simulink model "Classical_method"  (R2021a)
settings: Solver=VariableStepAuto  StartTime=0.0  StopTime=1400  RelTol=1e-3
values from neighbouring files (symbols this model uses):
  B = 0.029    [project.m]
  J = 0.1    [project.m]
  ke = 0.6    [project.m]
  kt = 0.6    [project.m]
  La = 1e-3    (= 0.001)    [project.m]
  Ra = 1    [project.m]
settings Model: SimulationMode=rapid-accelerator  Creator=User  LastModifiedBy=User
settings DataIOCC: ReturnWorkspaceOutputs=off

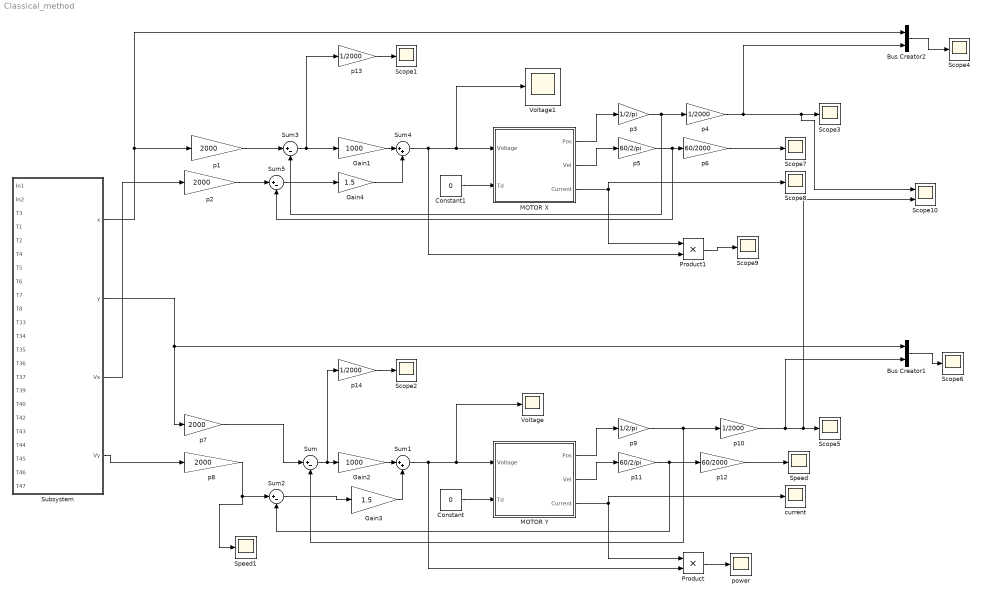
== system Classical_method ==
  Bus Creator1 : BusCreator  Inputs=2
  Bus Creator2 : BusCreator  Inputs=2
  Constant : Constant  Value=0
  Constant1 : Constant  Value=0
  Gain1 : Gain  Gain=1000
  Gain2 : Gain  Gain=1000
  Gain3 : Gain  Gain=1.5
  Gain4 : Gain  Gain=1.5
  MOTOR X : Subsystem
  MOTOR Y : Subsystem
  Product : Product
  Product1 : Product
  Scope{1..9} (9 alike) : Scope
  Scope10 : Scope  NumInputPorts=2
  Speed : Scope
  Speed1 : Scope
  Subsystem : Subsystem
  Sum{,2..3,5} (4 alike) : Sum  Inputs=|+-
  Sum1 : Sum  Inputs=|++
  Sum4 : Sum  Inputs=|++
  Voltage : Scope
  Voltage1 : Scope
  current : Scope
  p{1..2,7..8} (4 alike) : Gain  Gain=2000
  p{4,10,13..14} (4 alike) : Gain  Gain=1/2000
  p11 : Gain  Gain=60/2/pi
  p12 : Gain  Gain=60/2000
  p3 : Gain  Gain=1/2/pi
  p5 : Gain  Gain=60/2/pi
  p6 : Gain  Gain=60/2000
  p9 : Gain  Gain=1/2/pi
  power : Scope
  wires:
  MOTOR Y/1(Pos) -> p9/1
  p10/1 -> Bus Creator1/2, Scope10/2, Scope5/1
  Gain3/1 -> Sum1/2
  p5/1 -> Sum5/2, p6/1
  p7/1 -> Sum/1
  p3/1 -> Sum3/2, p4/1
  Constant1/1 -> MOTOR X/2(Td)
  MOTOR Y/3(Current) -> current/1, Product/1
  Sum5/1 -> Gain4/1
  Product1/1 -> Scope9/1
  Sum1/1 -> Product/2, Voltage/1, MOTOR Y/1(Voltage)
  p4/1 -> Bus Creator2/2, Scope10/1, Scope3/1
  Gain4/1 -> Sum4/2
  p12/1 -> Speed/1
  MOTOR X/3(Current) -> Scope8/1, Product1/1
  p8/1 -> Speed1/1, Sum2/1
  Bus Creator1/1 -> Scope6/1
  MOTOR X/2(Vel) -> p5/1
  Gain2/1 -> Sum1/1
  Gain1/1 -> Sum4/1
  Constant/1 -> MOTOR Y/2(Td)
  Product/1 -> power/1
  p6/1 -> Scope7/1
  Sum2/1 -> Gain3/1
  MOTOR Y/2(Vel) -> p11/1
  p2/1 -> Sum5/1
  Sum3/1 -> p13/1, Gain1/1
  p11/1 -> Sum2/2, p12/1
  Sum4/1 -> Product1/2, Voltage1/1, MOTOR X/1(Voltage)
  Sum/1 -> p14/1, Gain2/1
  Subsystem/2(y) -> Bus Creator1/1, p7/1
  Subsystem/3(Vx) -> p2/1
  p9/1 -> Sum/2, p10/1
  Subsystem/4(Vy) -> p8/1
  MOTOR X/1(Pos) -> p3/1
  Subsystem/1(x) -> p1/1, Bus Creator2/1
  Bus Creator2/1 -> Scope4/1
  p13/1 -> Scope1/1
  p14/1 -> Scope2/1
  p1/1 -> Sum3/1

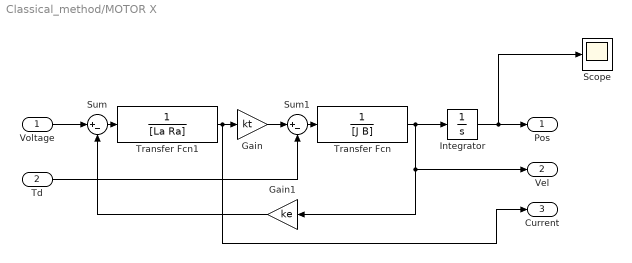
== system Classical_method/MOTOR X ==
  Voltage : Inport
  Td : Inport  Port=2
  Gain : Gain  Gain=kt
  Gain1 : Gain  Gain=ke
  Integrator : Integrator  InitialCondition=12000*pi
  Scope : Scope
  Sum : Sum  Inputs=|+-
  Sum1 : Sum  Inputs=|+-
  Transfer Fcn : TransferFcn  Denominator=[J B]
  Transfer Fcn1 : TransferFcn  Denominator=[La Ra]
  Pos : Outport  VectorParamsAs1DForOutWhenUnconnected=off
  Vel : Outport  Port=2  VectorParamsAs1DForOutWhenUnconnected=off
  Current : Outport  Port=3  VectorParamsAs1DForOutWhenUnconnected=off
  wires:
  Integrator/1 -> Scope/1, Pos/1
  Voltage/1 -> Sum/1
  Transfer Fcn/1 -> Integrator/1, Vel/1, Gain1/1
  Sum1/1 -> Transfer Fcn/1
  Td/1 -> Sum1/2
  Gain1/1 -> Sum/2
  Sum/1 -> Transfer Fcn1/1
  Transfer Fcn1/1 -> Current/1, Gain/1
  Gain/1 -> Sum1/1

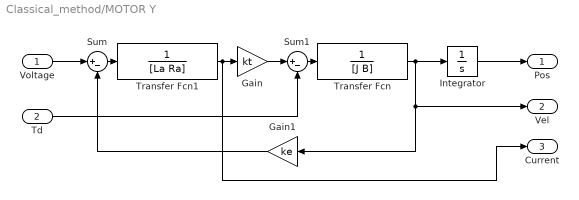
== system Classical_method/MOTOR Y ==
  Voltage : Inport
  Td : Inport  Port=2
  Gain : Gain  Gain=kt
  Gain1 : Gain  Gain=ke
  Integrator : Integrator  InitialCondition=8000*pi
  Sum : Sum  Inputs=|+-
  Sum1 : Sum  Inputs=|+-
  Transfer Fcn : TransferFcn  Denominator=[J B]
  Transfer Fcn1 : TransferFcn  Denominator=[La Ra]
  Pos : Outport  VectorParamsAs1DForOutWhenUnconnected=off
  Vel : Outport  Port=2  VectorParamsAs1DForOutWhenUnconnected=off
  Current : Outport  Port=3  VectorParamsAs1DForOutWhenUnconnected=off
  wires:
  Integrator/1 -> Pos/1
  Voltage/1 -> Sum/1
  Transfer Fcn/1 -> Integrator/1, Vel/1, Gain1/1
  Sum1/1 -> Transfer Fcn/1
  Td/1 -> Sum1/2
  Gain1/1 -> Sum/2
  Sum/1 -> Transfer Fcn1/1
  Transfer Fcn1/1 -> Current/1, Gain/1
  Gain/1 -> Sum1/1

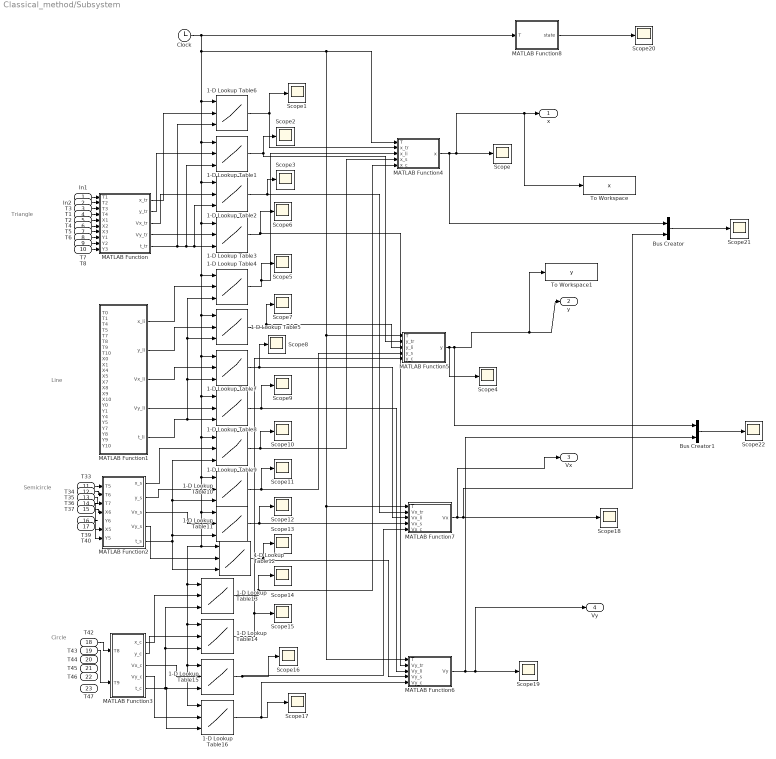
== system Classical_method/Subsystem ==
  note: Circle
  note: Semicircle
  note: Line
  note: Triangle
  In1 : Inport
  In2 : Inport  Port=2
  T3 : Inport  Port=3
  T1 : Inport  Port=4
  T2 : Inport  Port=5
  T4 : Inport  Port=6
  T5 : Inport  Port=7
  T6 : Inport  Port=8
  T7 : Inport  Port=9
  T8 : Inport  Port=10
  T33 : Inport  Port=11
  T34 : Inport  Port=12
  T35 : Inport  Port=13
  T36 : Inport  Port=14
  T37 : Inport  Port=15
  T39 : Inport  Port=16
  T40 : Inport  Port=17
  T42 : Inport  Port=18
  T43 : Inport  Port=19
  T44 : Inport  Port=20
  T45 : Inport  Port=21
  T46 : Inport  Port=22
  T47 : Inport  Port=23
  1-D Lookup Table{1..16} (16 alike) : Lookup_n-D  NumberOfTableDimensions=1  BreakpointsForDimension1Source=Input port  BreakpointsForDimension1=[-5:5]  TableSource=Input port  Table=tanh([-5:5])  InternalRulePriority=Speed  RndMeth=Simplest  InputSameDT=on
      settings: InputPortMap=u0,p221,p5
  Bus Creator : BusCreator  Inputs=2
  Bus Creator1 : BusCreator  Inputs=2
  Clock : Clock
  MATLAB Function : MATLAB Function  TreatAsAtomicUnit=on
  MATLAB Function1 : MATLAB Function  TreatAsAtomicUnit=on
  MATLAB Function2 : MATLAB Function  TreatAsAtomicUnit=on
  MATLAB Function3 : MATLAB Function  TreatAsAtomicUnit=on
  MATLAB Function4 : MATLAB Function  TreatAsAtomicUnit=on
  MATLAB Function5 : MATLAB Function  TreatAsAtomicUnit=on
  MATLAB Function6 : MATLAB Function  TreatAsAtomicUnit=on
  MATLAB Function7 : MATLAB Function  TreatAsAtomicUnit=on
  MATLAB Function8 : MATLAB Function  TreatAsAtomicUnit=on
  Scope{,1..22} (23 alike) : Scope
  To Workspace : ToWorkspace  VariableName=x  SampleTime=-1
  To Workspace1 : ToWorkspace  VariableName=y  SampleTime=-1
  x : Outport
  y : Outport  Port=2
  Vx : Outport  Port=3
  Vy : Outport  Port=4
  wires:
  Clock/1 -> MATLAB Function8/1(T), MATLAB Function6/1(T), MATLAB Function7/1(T), MATLAB Function5/1(T), MATLAB Function4/1(T), 1-D Lookup Table6/1, 1-D Lookup Table1/1, 1-D Lookup Table2/1, 1-D Lookup Table3/1, 1-D Lookup Table16/1, 1-D Lookup Table15/1, 1-D Lookup Table14/1, 1-D Lookup Table13/1, 1-D Lookup Table12/1, 1-D Lookup Table11/1, 1-D Lookup Table10/1, 1-D Lookup Table9/1, 1-D Lookup Table8/1, 1-D Lookup Table7/1, 1-D Lookup Table5/1, 1-D Lookup Table4/1
  1-D Lookup Table6/1 -> Scope1/1, MATLAB Function4/2(x_tr)
  1-D Lookup Table1/1 -> MATLAB Function5/2(y_tr), Scope2/1
  1-D Lookup Table2/1 -> MATLAB Function7/2(Vx_tr), Scope3/1
  1-D Lookup Table4/1 -> MATLAB Function4/3(x_li), Scope5/1
  1-D Lookup Table7/1 -> Scope8/1, MATLAB Function7/3(Vx_li)
  1-D Lookup Table8/1 -> MATLAB Function6/3(Vy_li), Scope9/1
  1-D Lookup Table9/1 -> MATLAB Function4/4(x_s), Scope10/1
  1-D Lookup Table10/1 -> MATLAB Function5/4(y_s), Scope11/1
  1-D Lookup Table11/1 -> MATLAB Function7/4(Vx_s), Scope12/1
  1-D Lookup Table12/1 -> MATLAB Function6/4(Vy_s), Scope13/1
  1-D Lookup Table13/1 -> MATLAB Function4/5(x_c), Scope14/1
  1-D Lookup Table15/1 -> MATLAB Function7/5(Vx_c), Scope16/1
  1-D Lookup Table16/1 -> MATLAB Function6/5(Vy_c), Scope17/1
  In1/1 -> MATLAB Function/1(T1)
  In2/1 -> MATLAB Function/2(T2)
  T3/1 -> MATLAB Function/3(T3)
  T1/1 -> MATLAB Function/4(T4)
  T2/1 -> MATLAB Function/5(X1)
  T4/1 -> MATLAB Function/6(X2)
  T5/1 -> MATLAB Function/7(X3)
  T6/1 -> MATLAB Function/8(Y1)
  T7/1 -> MATLAB Function/9(Y2)
  T8/1 -> MATLAB Function/10(Y3)
  T33/1 -> MATLAB Function2/1(T5)
  T34/1 -> MATLAB Function2/2(T6)
  T35/1 -> MATLAB Function2/3(T7)
  T36/1 -> MATLAB Function2/6(X5)
  T37/1 -> MATLAB Function2/4(X6)
  T39/1 -> MATLAB Function2/7(Y5)
  T42/1 -> MATLAB Function3/1(T8)
  T43/1 -> MATLAB Function3/2(T9)
  1-D Lookup Table14/1 -> MATLAB Function5/5(y_c), Scope15/1
  MATLAB Function1/1(x_li) -> 1-D Lookup Table4/2
  MATLAB Function1/2(y_li) -> 1-D Lookup Table5/2
  MATLAB Function1/3(Vx_li) -> 1-D Lookup Table7/2
  MATLAB Function1/4(Vy_li) -> 1-D Lookup Table8/2
  MATLAB Function1/5(t_li) -> 1-D Lookup Table4/3, 1-D Lookup Table5/3, 1-D Lookup Table7/3, 1-D Lookup Table8/3
  MATLAB Function2/5(t_s) -> 1-D Lookup Table11/3, 1-D Lookup Table10/3, 1-D Lookup Table9/3, 1-D Lookup Table12/3
  MATLAB Function3/5(t_c) -> 1-D Lookup Table14/3, 1-D Lookup Table13/3, 1-D Lookup Table16/3, 1-D Lookup Table15/3
  MATLAB Function2/1(x_s) -> 1-D Lookup Table9/2
  MATLAB Function2/2(y_s) -> 1-D Lookup Table10/2
  MATLAB Function2/3(Vx_s) -> 1-D Lookup Table11/2
  MATLAB Function2/4(Vy_s) -> 1-D Lookup Table12/2
  MATLAB Function3/1(x_c) -> 1-D Lookup Table13/2
  MATLAB Function3/2(y_c) -> 1-D Lookup Table14/2
  MATLAB Function3/3(Vx_c) -> 1-D Lookup Table15/2
  MATLAB Function3/4(Vy_c) -> 1-D Lookup Table16/2
  MATLAB Function/5(t_tr) -> 1-D Lookup Table6/3, 1-D Lookup Table1/3, 1-D Lookup Table2/3, 1-D Lookup Table3/3
  MATLAB Function/1(x_tr) -> 1-D Lookup Table6/2
  MATLAB Function/2(y_tr) -> 1-D Lookup Table1/2
  MATLAB Function/3(Vx_tr) -> 1-D Lookup Table2/2
  MATLAB Function/4(Vy_tr) -> 1-D Lookup Table3/2
  1-D Lookup Table5/1 -> Scope7/1, MATLAB Function5/3(y_li)
  1-D Lookup Table3/1 -> MATLAB Function6/2(Vy_tr), Scope6/1
  MATLAB Function8/1(state) -> Scope20/1
  Bus Creator/1 -> Scope21/1
  Bus Creator1/1 -> Scope22/1
  MATLAB Function4/1(x) -> Bus Creator/1, To Workspace/1, x/1, Scope/1
  MATLAB Function5/1(y) -> Scope4/1, To Workspace1/1, y/1, Bus Creator1/1
  MATLAB Function7/1(Vx) -> Vx/1, Scope18/1, Bus Creator/2
  MATLAB Function6/1(Vy) -> Bus Creator1/2, Vy/1, Scope19/1

== matlab function Classical_method/Subsystem/MATLAB Function3 ==
  data: x_c output; T8 input; T9 input; y_c output; Vx_c output; Vy_c output; t_c output
function [x_c,y_c,Vx_c,Vy_c,t_c] = fcn(T8,T9)
T8=1005;
T9=1285;
t=T8:0.1:T9;
sigma=(t-T8)/(T9-T8);
lambda=poly5(sigma);
theta=lambda*2*pi;
R=0.5;
P=R*[cos(theta);sin(theta)];
x8=P(1,:)+2.25;
y8=P(2,:)+1;
lambdavel=poly5d(sigma);
Vx8=2*R*pi/(T9-T8)*lambdavel.*[-sin(theta)];
Vy8=2*R*pi/(T9-T8)*lambdavel.*[cos(theta)];
x_c=x8;
y_c=y8;
t_c=T8+sigma*(T9-T8);
Vx_c=Vx8;
Vy_c=Vy8;

== matlab function Classical_method/Subsystem/MATLAB Function4 ==
  data: T input; x output; x_tr input; x_li input; x_s input; x_c input
function x = fcn(T,x_tr,x_li,x_s,x_c)
if T>=260 && T<=530
    x=x_tr
elseif T>=675 && T<=905
    x=x_s
elseif T>=1005 && T<=1285
    x=x_c
else
    x=x_li
end

== matlab function Classical_method/Subsystem/MATLAB Function5 ==
  data: T input; y output; y_tr input; y_li input; y_s input; y_c input
function y = fcn(T,y_tr,y_li,y_s,y_c)
if T>=260 && T<=530
    y=y_tr
elseif T>=675 && T<=905
    y=y_s
elseif T>=1005 && T<=1285
    y=y_c
else
    y=y_li
end

== matlab function Classical_method/Subsystem/MATLAB Function6 ==
  data: T input; Vy output; Vy_tr input; Vy_li input; Vy_s input; Vy_c input
function Vy = fcn(T,Vy_tr,Vy_li,Vy_s,Vy_c)
if T>=260 && T<=530
    Vy=Vy_tr
elseif T>=675 && T<=905
    Vy=Vy_s
elseif T>=1005 && T<=1285
    Vy=Vy_c
else
    Vy=Vy_li
end

== matlab function Classical_method/Subsystem/MATLAB Function7 ==
  data: T input; Vx output; Vx_tr input; Vx_li input; Vx_s input; Vx_c input
function Vx = fcn(T,Vx_tr,Vx_li,Vx_s,Vx_c)
if T>=260 && T<=530
    Vx=Vx_tr
elseif T>=675 && T<=905
    Vx=Vx_s
elseif T>=1005 && T<=1285
    Vx=Vx_c
else
    Vx=Vx_li
end

== matlab function Classical_method/Subsystem/MATLAB Function8 ==
  data: T input; state output
function state = fcn(T)
if T>=260 && T<=530
    state=true
elseif T>=675 && T<=905
    state=true
elseif T>=1005 && T<=1285
    state=true
else
    state=false
end

== matlab function Classical_method/Subsystem/MATLAB Function1 ==
  data: T0 input; x_li output; T1 input; T4 input; T5 input; T7 input; T8 input; T9 input; T10 input; X0 input; X1 input; X4 input; X5 input; X7 input; X8 input; X9 input; X10 input; Y0 input; Y1 input; y_li output; Vx_li output; Vy_li output; t_li output; Y4 input; Y5 input; Y7 input; Y8 input; Y9 input; Y10 input
function [x_li,y_li,Vx_li,Vy_li,t_li] = fcn(T0,T1,T4,T5,T7,T8,T9,T10,X0,X1,X4,X5,X7,X8,X9,X10,Y0,Y1,Y4,Y5,Y7,Y8,Y9,Y10)
T0=0;
T1=260;
T4=530;
T5=675;
T7=905;
T8=1005;
T9=1285;
T10=1400;
X1=0.5;
X4=0.5;
X0=3;
Y0=2;
X5=1.75;
X7=1.75;
Y5=1.5;
Y7=1.5;
X8=2.75;
X9=2.75;
X10=3;
Y10=2;
Y8=1;
Y9=1;
Y1=0.5;
Y4=0.5;
sigma=0.01:0.01:1;
t0=T0+sigma*(T1-T0);
t4=T4+sigma*(T5-T4);
t7=T7+sigma*(T8-T7);
t9=T9+sigma*(T10-T9);
t_li=[t0 t4 t7 t9];
lambda=poly5(sigma);
x0=X0+lambda*(X1-X0);
x4=X4+lambda*(X5-X4);
x7=X7+lambda*(X8-X7);
x9=X9+lambda*(X10-X9);
x_li=[x0 x4 x7 x9];
y0=Y0+lambda*(Y1-Y0);
y4=Y4+lambda*(Y5-Y4);
y7=Y7+lambda*(Y8-Y7);
y9=Y9+lambda*(Y10-Y9);
y_li=[y0 y4 y7 y9];
lambdavel=poly5d(sigma);
Vx0=(X1-X0)/(T1-T0).*lambdavel;
Vx4=(X5-X4)/(T5-T4).*lambdavel;
Vx7=(X8-X7)/(T8-T7).*lambdavel;
Vx9=(X10-X9)/(T10-T9).*lambdavel;
Vy0=(Y1-Y0)/(T1-T0).*lambdavel;
Vy4=(Y5-Y4)/(T5-T4).*lambdavel;
Vy7=(Y8-Y7)/(T8-T7).*lambdavel;
Vy9=(Y10-Y9)/(T10-T9).*lambdavel;
Vx_li=[Vx0 Vx4 Vx7 Vx9];
Vy_li=[Vy0 Vy4 Vy7 Vy9];

== matlab function Classical_method/Subsystem/MATLAB Function ==
  data: T1 input; x_tr output; T2 input; T3 input; T4 input; X1 input; X2 input; X3 input; Y1 input; Y2 input; Y3 input; y_tr output; Vx_tr output; Vy_tr output; t_tr output
function [x_tr,y_tr,Vx_tr,Vy_tr,t_tr] = fcn(T1,T2,T3,T4,X1,X2,X3,Y1,Y2,Y3)
T1=260;
T2=330;
T3=460;
T4=530;
X1=0.5;
X2=1.25;
X3=0.25;
Y1=0.5;
Y2=0.25;
Y3=1.25;
sigma=0.01:0.01:1;
t1=T1+sigma*(T2-T1);
t2=T2+sigma*(T3-T2);
t3=T3+sigma*(T4-T3);
t_tr=[t1 t2 t3];
lambda=poly5(sigma);
x1=X1+lambda*(X2-X1);
x2=X2+lambda*(X3-X2);
x3=X3+lambda*(X1-X3);
y1=Y1+lambda*(Y2-Y1);
y2=Y2+lambda*(Y3-Y2);
y3=Y3+lambda*(Y1-Y3);
lambdavel=poly5d(sigma);
Vx1=(X2-X1)/(T2-T1).*lambdavel;
Vx2=(X3-X2)/(T3-T2).*lambdavel;
Vx3=(X1-X3)/(T4-T3).*lambdavel;
Vy1=(Y2-Y1)/(T2-T1).*lambdavel;
Vy2=(Y3-Y2)/(T3-T2).*lambdavel;
Vy3=(Y1-Y3)/(T4-T3).*lambdavel;
x_tr=[x1 x2 x3];
y_tr=[y1 y2 y3];
Vx_tr=[Vx1 Vx2 Vx3];
Vy_tr=[Vy1 Vy2 Vy3];

== matlab function Classical_method/Subsystem/MATLAB Function2 ==
  data: x_s output; T5 input; T6 input; T7 input; X6 input; Y6 input; X5 input; Y5 input; y_s output; Vx_s output; Vy_s output; t_s output
function [x_s,y_s,Vx_s,Vy_s,t_s] = fcn(T5,T6,T7,X6,Y6,X5,Y5)
T5=675;
T6=815;
T7=905;
X6=0.75;
X5=1.75;
Y6=1.5;
Y5=1.5;
t5=T5:0.1:T6;
sigm=(t5-T5)/(T6-T5);
lambda=poly5(sigm);
theta=lambda*pi;
R=0.5;
P=R*[cos(theta);sin(theta)];
x5=P(1,:)+1.25;
y5=P(2,:)+1.5;
lambdavel=poly5d(sigm);
Vx5=R*[-sin(theta)]*2*pi/(T6-T5).*lambdavel;
Vy5=R*[cos(theta)]*2*pi/(T6-T5).*lambdavel;
sigma=0.01:0.01:1;
t6=T6+sigma*(T7-T6);
lambda=poly5(sigma);
x6=X6+lambda*(X5-X6);
y6=Y6+lambda*(Y5-Y6);
lambdavel=poly5d(sigma);
Vx6=(X5-X6)/(T7-T6).*lambdavel;
Vy6=(Y5-Y6)/(T7-T6).*lambdavel;
x_s=[x5 x6];
y_s=[y5 y6];
Vx_s=[Vx5 Vx6];
Vy_s=[Vy5 Vy6];
t_s=[t5 t6];
